simulink model "quanser"  (R2022b)
settings: Solver=ode1  StartTime=0.0  StopTime=6  FixedStep=0.002  RelTol=1e-3
libraries: robotlib x5
settings Model: Creator=guillermo  LastModifiedBy=guillermo

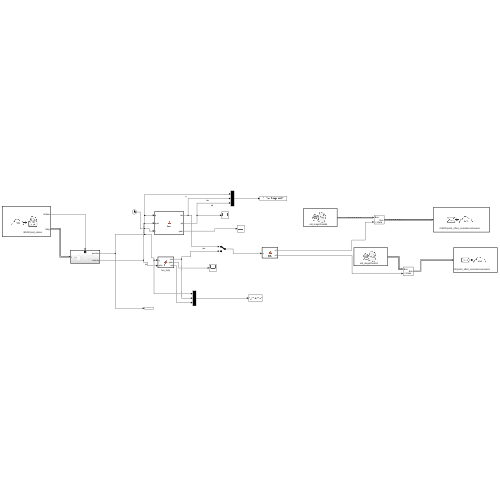
[thumbnail: Simulink's stored preview of the top-level diagram]
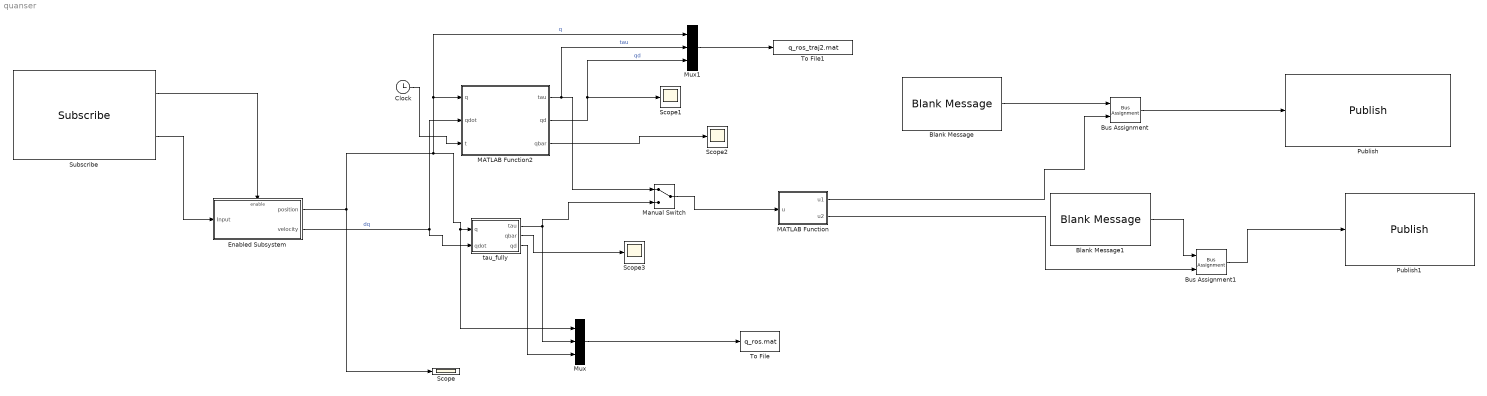
== system quanser ==
  Blank Message : robotlib/Blank Message  messageClass=Message  entityType=std_msgs/Float64  messageType=std_msgs/Float64  SampleTime=inf  legacyBusStruct=off
      settings: LibrarySourceBlock=roslib/ROS/Blank Message
  Blank Message1 : robotlib/Blank Message  messageClass=Message  entityType=std_msgs/Float64  messageType=std_msgs/Float64  SampleTime=inf  legacyBusStruct=off
      settings: LibrarySourceBlock=roslib/ROS/Blank Message
  Bus Assignment : BusAssignment  AssignedSignals=Data
  Bus Assignment1 : BusAssignment  AssignedSignals=Data
  Clock : Clock
  Enabled Subsystem : Subsystem  TreatAsAtomicUnit=on
  MATLAB Function : MATLAB Function  TreatAsAtomicUnit=on
  MATLAB Function2 : MATLAB Function  TreatAsAtomicUnit=on
  Manual Switch : ManualSwitch
  Mux : Mux  Inputs=3
  Mux1 : Mux  Inputs=3
  Publish : robotlib/Publish  topicSource=Select from ROS network  topic=/SDOF/joint1_effort_controller/command  messageType=std_msgs/Float64  legacyBusStruct=off  messageQueueLength=1
      settings: LibrarySourceBlock=roslib/ROS/Publish
  Publish1 : robotlib/Publish  topicSource=Select from ROS network  topic=/SDOF/joint2_effort_controller/command  messageType=std_msgs/Float64  legacyBusStruct=off  messageQueueLength=1
      settings: LibrarySourceBlock=roslib/ROS/Publish
  Scope{,1..3} (4 alike) : Scope
  Subscribe : robotlib/Subscribe  topicSource=Select from ROS network  topic=/SDOF/joint_states  messageType=sensor_msgs/JointState  SampleTime=-1  legacyBusStruct=off  messageQueueLength=1
      settings: LibrarySourceBlock=roslib/ROS/Subscribe
  To File : ToFile  Filename=q_ros.mat  MatrixName=q  SaveFormat=Timeseries
  To File1 : ToFile  Filename=q_ros_traj2.mat  MatrixName=q  SaveFormat=Timeseries
  "tau_fully " : MATLAB Function  TreatAsAtomicUnit=on
  wires:
  MATLAB Function/1(u1) -> Bus Assignment/2
  Manual Switch/1 -> MATLAB Function/1(u)
  Enabled Subsystem/2(velocity) -> MATLAB Function2/2(qdot), "tau_fully "/2(qdot)  "dq"
  MATLAB Function/2(u2) -> Bus Assignment1/2
  Bus Assignment1/1 -> Publish1/1
  Blank Message/1 -> Bus Assignment/1
  Bus Assignment/1 -> Publish/1
  Blank Message1/1 -> Bus Assignment1/1
  Subscribe/1 -> Enabled Subsystem/Enable
  Subscribe/2 -> Enabled Subsystem/1(Input)
  Enabled Subsystem/1(position) -> Mux/1, "tau_fully "/1(q), Mux1/1, MATLAB Function2/1(q), Scope/1  "q"
  "tau_fully "/1(tau) -> Manual Switch/2, Mux/2
  Clock/1 -> MATLAB Function2/3(t)
  MATLAB Function2/3(qbar) -> Scope2/1
  "tau_fully "/2(qbar) -> Scope3/1
  "tau_fully "/3(qd) -> Mux/3
  Mux/1 -> To File/1
  Mux1/1 -> To File1/1
  MATLAB Function2/1(tau) -> Mux1/2, Manual Switch/1  "tau"
  MATLAB Function2/2(qd) -> Scope1/1, Mux1/3  "qd"

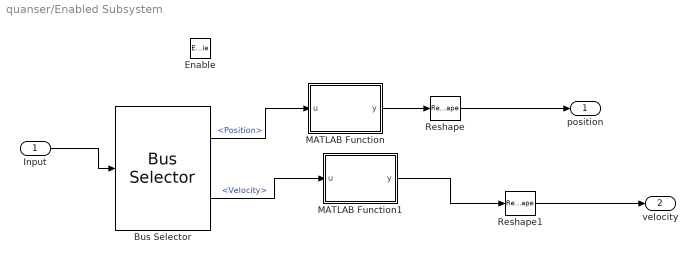
== system quanser/Enabled Subsystem ==
  Input : Inport
  Enable : EnablePort
  Bus Selector : BusSelector  OutputSignals=Position,Velocity
  MATLAB Function : MATLAB Function  TreatAsAtomicUnit=on
  MATLAB Function1 : MATLAB Function  TreatAsAtomicUnit=on
  Reshape : Reshape  OutputDimensionality=Column vector (2-D)
  Reshape1 : Reshape  OutputDimensionality=Column vector (2-D)
  position : Outport
  velocity : Outport  Port=2
  wires:
  Input/1 -> Bus Selector/1
  Bus Selector/1 -> MATLAB Function/1(u)  "<Position>"
  Bus Selector/2 -> MATLAB Function1/1(u)  "<Velocity>"
  MATLAB Function/1(y) -> Reshape/1
  MATLAB Function1/1(y) -> Reshape1/1
  Reshape/1 -> position/1
  Reshape1/1 -> velocity/1

== matlab function quanser/tau_fully  ==
  data: q input; qdot input; tau output size=[2 1]; qbar output; qd output
function [tau,qbar,qd]= fcn(q,qdot)
qd=[0.6;0.8];
qbar=q-qd;
q2=q(2);

%Conversion constants from A to Nm ([Nm/A]) obtained from feedback example
%Ktg1=8.9250;
%Ktg2=0.87;
Ktg1=1;
Ktg2=0.6;


Kp=diag([6,2])*1;
Ki=diag([30,10]);
Kd=diag([0.5,0.1]);
%Mass Inertial matrix
m1=1.5;
m2=0.8733;
I1=0.0102;
I2=0.0085;
r1=0.159;
r2=0.0550; 
l1=0.3493;
l2=0.2975;
a1=m1*r1^2+m2*l1^2+I1;
a2=m2*r2^2+I2;
b=m2*l1*r2;
M=[a1+a2+2*b*cos(q2) a2+b*cos(q2); a2+b*cos(q2) a2];

p=M*qdot;
p1=p(1);
p2=p(2);

%% For the kinetic shaping
dMdq2=(1/(a1*a2 - b^2*cos(q2)^2)^2)*[-(2*a2*b^2*cos(q2)*sin(q2)), (b*sin(q2)*(a1*a2 + b^2*cos(q2)^2 + 2*a2*b*cos(q2)));
(b*sin(q2)*(a1*a2 + b^2*cos(q2)^2 + 2*a2*b*cos(q2))),-(2*b*sin(q2)*(a1 + b*cos(q2))*(a2 + b*cos(q2)))];
big_K=eye(2)+Kd*inv(M);
nablaH=[[0;[p1 p2]*dMdq2*[p1;p2]];inv(M)*[p1; p2]];
nabla_y=[0,0;...
    (b*p2*sin(q2))/(a1*a2 - b^2*cos(q2)^2) + (2*b^2*p2*cos(q2)*sin(q2)*(a2 + b*cos(q2)))/(a1*a2 - b^2*cos(q2)^2)^2 - (2*a2*b^2*p1*cos(q2)*sin(q2))/(a1*a2 - b^2*cos(q2)^2)^2, (b*p1*sin(q2))/(a1*a2 - b^2*cos(q2)^2) - (2*b*p2*sin(q2))/(a1*a2 - b^2*cos(q2)^2) - (2*b^2*p2*cos(q2)*sin(q2)*(a1 + a2 + 2*b*cos(q2)))/(a1*a2 - b^2*cos(q2)^2)^2 + (2*b^2*p1*cos(q2)*sin(q2)*(a2 + b*cos(q2)))/(a1*a2 - b^2*cos(q2)^2)^2];
ks=-Kd*[-inv(M), nabla_y']*nablaH;

%% Potential shaping and Damping injection
ps=-Ki*qbar;
di=-Kp*qdot;

%% Controller
tau=inv(big_K)*(ps+di+ks);
%tau= [1/Ktg1 0;0 1/Ktg2]*tau_torque; %Conversion to current
end

== matlab function quanser/MATLAB Function2 ==
  data: q input; tau output; qdot input; t input; qd output; qbar output
function [tau,qd,qbar]= fcn(q,qdot,t)
qd=[0.6;0.8];
meat_trajectory_q1_4=[ -0.0399    0.3374   -0.8211    1.0209   -1.2782];
meat_trajectory_q2_4=[0.0673   -0.5507    1.2833   -1.2111    1.1745];
meat_trajectory_q1_6_10=[-0.000009277410992   0.000090314572996   0.001297915318347  -0.026304684172646   0.182139231267472  -0.651240398320963 1.291186157873882  -1.351097352337477   0.532389548502892 0.337857208231721  -1.153099673342133];
meat_trajectory_q2_6_10=[    0.000017923804761  -0.000205193188962  -0.001724084705260  0.042647029822475  -0.306877336120589   1.117504651378960 -2.250235814246918   2.429646337439796  -1.119318576516060 -0.159123191836711   1.021578886099627 ];

meat_q1= polyval(meat_trajectory_q1_6_10,t);
meat_q2= polyval(meat_trajectory_q2_6_10,t);
qd = [meat_q1;meat_q2];



qbar=q-qd;%q position receiveed qd-position desired
q2=q(2);

%Conversion constants from A to Nm ([Nm/A]) obtained from feedback example
%Ktg1=8.9250;
%Ktg2=0.87;
Ktg1=1;
Ktg2=0.6;


Kp=diag([3.5,1.74])*1;

Ki=diag([30,10]);
Kd=diag([0.1,0.1]);
%Mass Inertial matrix
m1=1.5;
m2=0.8733;
I1=0.0102;
I2=0.0085;
r1=0.159;
r2=0.0550; 
l1=0.3493;
l2=0.2975;
a1=m1*r1^2+m2*l1^2+I1;
a2=m2*r2^2+I2;
b=m2*l1*r2;
M=[a1+a2+2*b*cos(q2) a2+b*cos(q2); a2+b*cos(q2) a2];

p=M*qdot;
p1=p(1);
p2=p(2);

%% For the kinetic shaping
dMdq2=(1/(a1*a2 - b^2*cos(q2)^2)^2)*[-(2*a2*b^2*cos(q2)*sin(q2)), (b*sin(q2)*(a1*a2 + b^2*cos(q2)^2 + 2*a2*b*cos(q2)));
(b*sin(q2)*(a1*a2 + b^2*cos(q2)^2 + 2*a2*b*cos(q2))),-(2*b*sin(q2)*(a1 + b*cos(q2))*(a2 + b*cos(q2)))];
big_K=eye(2)+Kd*inv(M);
nablaH=[[0;[p1 p2]*dMdq2*[p1;p2]];inv(M)*[p1; p2]];
nabla_y=[0,0;...
    (b*p2*sin(q2))/(a1*a2 - b^2*cos(q2)^2) + (2*b^2*p2*cos(q2)*sin(q2)*(a2 + b*cos(q2)))/(a1*a2 - b^2*cos(q2)^2)^2 - (2*a2*b^2*p1*cos(q2)*sin(q2))/(a1*a2 - b^2*cos(q2)^2)^2, (b*p1*sin(q2))/(a1*a2 - b^2*cos(q2)^2) - (2*b*p2*sin(q2))/(a1*a2 - b^2*cos(q2)^2) - (2*b^2*p2*cos(q2)*sin(q2)*(a1 + a2 + 2*b*cos(q2)))/(a1*a2 - b^2*cos(q2)^2)^2 + (2*b^2*p1*cos(q2)*sin(q2)*(a2 + b*cos(q2)))/(a1*a2 - b^2*cos(q2)^2)^2];
ks=-Kd*[-inv(M), nabla_y']*nablaH;

%% Potential shaping and Damping injection
ps=-Ki*qbar;
di=-Kp*qdot;

%% Controller
tau=inv(big_K)*(ps+di+ks);
end

== matlab function quanser/MATLAB Function ==
  data: u input; u1 output; u2 output
function [u1,u2]= fcn(u)
u1=u(1)
u2=u(2)

== matlab function quanser/Enabled Subsystem/MATLAB Function ==
  data: u input; y output
function y = fcn(u)
y=[0;0]

y(1)=u(1)
y(2)=u(2)

== matlab function quanser/Enabled Subsystem/MATLAB Function1 ==
  data: u input; y output
function y = fcn(u)
y=[0;0]

y(1)=u(1)
y(2)=u(2)
